simulink model "PTB_ConventionalModel"  (R2018a)
settings: Solver=ode23t  StartTime=0.0  StopTime=TimeUS06  RelTol=1e-3
model workspace (MAT data in the model file):
  Af = 4
  Cd = 0.3
  D = 0.322411602927
  DownShiftSpeeds = [11.05 18.7 28.9 38.675 51.425 11.05 18.7 28.9 38.675 51.425 11.05 18.7 ... (85 elements, 5x17)]
  DrCycles : struct (value not decoded)
  I = 0.25
  Kbr = 10000
  P = 15
  PedalPositions = [0 6.2485 12.4969 18.7454 24.9939 31.2424 37.4908 43.7393 49.9878 56.2363 62.4847 68.7332 ... (17 elements, 1x17)]
  TimeHWFET = 765
  TimeUDDS = 1372
  TimeUS06 = 596
  UpShiftSpeeds = [12.75 20.997635 31.45 42.16136 55.58864 12.75 20.997635 31.45 42.16136 55.58864 12.75 20.997635 ... (85 elements, 5x17)]
  axle_b = 10
  axle_k = 5000
  convAxle_wc = 500
  diffRatio = 3.4
  driveshaft_b = 10
  driveshaft_k = 2500
  driveshaft_wc = 500
  engineSpeedPoints_rpm = [750 1053.57142857 1357.14285714 1660.71428571 1964.28571429 2267.85714286 2571.42857143 2875 3178.57142857 3482.14285714 3785.71428571 4089.28571429 ... (15 elements, 1x15)]
  engineTorqueMap_Nm = [-13.6738264269 15.0034460821 26.4289521305 37.8539339756 49.2854604964 60.7146317399 72.0173711595 77.7345012802 77.7345012802 77.7345012802 77.7345012802 77.7345012802 ... (240 elements, 16x15)]
  engineTorquePoints_Nm = [0 15 26.4285714286 37.8571428571 49.2857142857 60.7142857143 72.1428571429 83.5714285714 95 106.428571429 117.857142857 129.285714286 ... (16 elements, 1x16)]
  vehicleMass = 1500
  wheelRadius = 0.35
libraries: Wheels_Driver_VehDyn_Lib x3, autolibsharedcoupling x2, simulink x2, autolibshareddiff x1, autolibsharedtransfixedgear x1, autolibenginesystems x1
(part 3 of 3)

== stateflow chart PTB_ConventionalModel/Driveline/Transmission/Transmission Shift Logic ==
  settings: updateMethod=DISCRETE  sampleTime=0.04
  state gear_state [parallel]
    settings: executionOrder=1
    state first
      entry:
      Gear = 1;
    state second
      entry:
      Gear = 2;
    state third
      entry:
      Gear = 3;
    state fourth
      entry:
      Gear = 4;
    state fifth
      entry:
      Gear = 5;
    state sixth
      entry:
      Gear = 6;
    (default) -> first
    second -> third [order 1] : UP
    first -> second : UP
    fourth -> fifth [order 1] : UP
    fifth -> sixth [order 1] : UP
    third -> fourth [order 1] : UP
    third -> second [order 2] : DOWN
    second -> first [order 2] : DOWN
    fifth -> fourth [order 2] : DOWN
    fourth -> third [order 2] : DOWN
    sixth -> fifth : DOWN
  state selection_state [parallel]
    du:[up_th]=calc_up(Gear,Throttle);
    du:[down_th]=calc_down(Gear,Throttle);
    settings: executionOrder=2
    state steady_state
    state upshifting
    state downshifting
    (default) -> steady_state
    steady_state -> upshifting [order 1] : [VehicleSpeed > up_th]
    steady_state -> downshifting [order 2] : [VehicleSpeed < down_th && Gear > 1]
    downshifting -> steady_state [order 1] : after(1,tick)
        | [VehicleSpeed <= down_th]
        | {gear_state.DOWN;}
    downshifting -> steady_state [order 2] : [VehicleSpeed > down_th]
    upshifting -> steady_state [order 1] : after(1,tick)
        | [VehicleSpeed >= up_th]
        | {gear_state.UP;}
    upshifting -> steady_state [order 2] : [VehicleSpeed < up_th]
  state up_th = calc_up(Gear,Throttle) [function]
  state down_th = calc_down(Gear,Throttle) [function]
  data: Gear function_input; Throttle function_input; up_th function_output; Gear function_input; Throttle function_input; down_th function_output; Throttle input double [0..100]; VehicleSpeed input double; Gear output double; down_th local double; up_th local double
  events: DOWN local EITHER_EDGE_EVENT; UP local EITHER_EDGE_EVENT
